simulink library "ROTH"  (R2016a)
settings: Solver=ode45  StartTime=0.0  StopTime=10.0  RelTol=1e-3
undefined symbols (not defined in the file): BUSY, CLEANED, EMPTY, FORWARD, GTSP, LEFT_BUSY_RIGHT_BUSY, LEFT_BUSY_RIGHT_CLEANED, LEFT_BUSY_RIGHT_EMPTY, LEFT_CLEANED_RIGHT_BUSY, LEFT_CLEANED_RIGHT_CLEANED, LEFT_CLEANED_RIGHT_EMPTY, LEFT_EMPTY_RIGHT_BUSY, LEFT_EMPTY_RIGHT_CLEANED, LEFT_EMPTY_RIGHT_EMPTY, MOVE_TURN_LEFT, MOVE_TURN_RIGHT, MOVE_U_TURN, MOVE_U_TURN_LEFT, MOVE_U_TURN_RIGHT, ROB_EAST, ROB_NORTH, ROB_SOUTH, ROB_WEST, STOP, UNCOVERED, ZIGZAG
settings Model: Creator=oelkawok  LastModifiedBy=oelkawok
settings DataIOCC: LimitDataPoints=on
settings DebuggingCC: AllowSymbolicDim=off

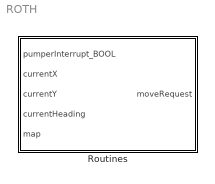
== system ROTH ==
  Routines : Subsystem

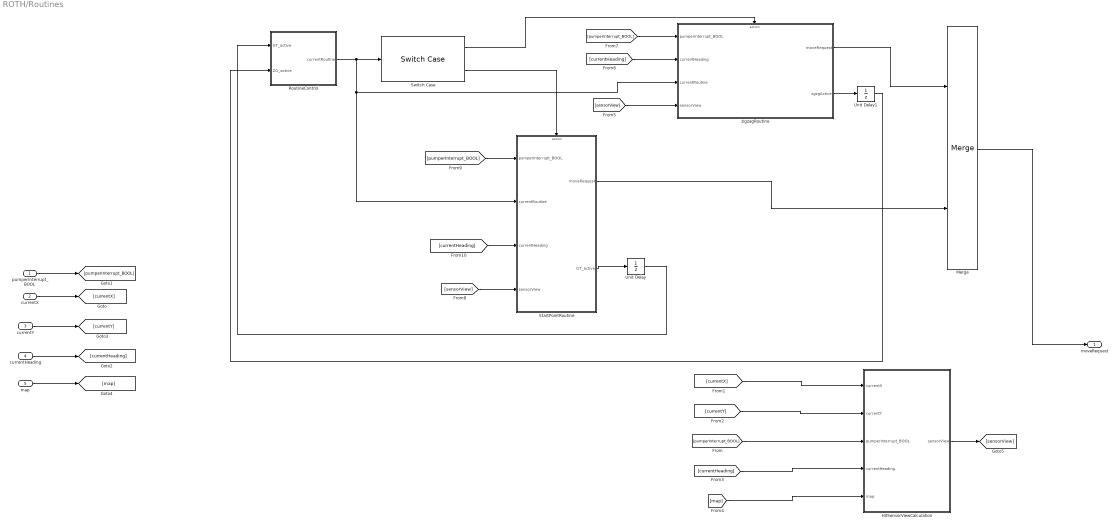
== system ROTH/Routines ==
  pumperInterrupt_BOOL : Inport
  currentX : Inport  Port=2
  currentY : Inport  Port=3
  currentHeading : Inport  Port=4
  map : Inport  Port=5
  HitSensorViewCalculation : Subsystem
  Merge : Merge
  RoutineControl : Subsystem
  StartPointRoutine : Subsystem
  Switch Case : SwitchCase  CaseConditions={ZIGZAG, GTSP}  ShowDefaultCase=off
      settings: AttributesFormatString=%<CaseConditions>
  Unit Delay : UnitDelay  InitialCondition=true  SampleTime=-1
  Unit Delay1 : UnitDelay  InitialCondition=false  SampleTime=-1
  zigzagRoutine : Subsystem
  moveRequest : Outport
  wires:
  [currentHeading] -> StartPointRoutine/3(currentHeading)
  [sensorView] -> StartPointRoutine/4(sensorView)
  [pumperInterrupt_BOOL] -> StartPointRoutine/1(pumperInterrupt_BOOL)
  Unit Delay1/1 -> RoutineControl/2(ZG_active)
  zigzagRoutine/2(zgzgActive) -> Unit Delay1/1
  zigzagRoutine/1(moveRequest) -> Merge/1
  StartPointRoutine/1(moveRequest) -> Merge/2
  [currentX] -> HitSensorViewCalculation/1(currentX)
  [currentY] -> HitSensorViewCalculation/2(currentY)
  [pumperInterrupt_BOOL] -> HitSensorViewCalculation/3(pumperInterrupt_BOOL)
  [currentHeading] -> HitSensorViewCalculation/4(currentHeading)
  [map] -> HitSensorViewCalculation/5(map)
  Switch Case/2 -> StartPointRoutine/Action
  Switch Case/1 -> zigzagRoutine/Action
  RoutineControl/1(currentRoutine) -> Switch Case/1, StartPointRoutine/2(currentRoutine), zigzagRoutine/3(currentRoutine)
  [currentHeading] -> zigzagRoutine/2(currentHeading)
  [pumperInterrupt_BOOL] -> zigzagRoutine/1(pumperInterrupt_BOOL)
  [sensorView] -> zigzagRoutine/4(sensorView)
  HitSensorViewCalculation/1(sensorView) -> [sensorView]
  Merge/1 -> moveRequest/1
  StartPointRoutine/2(GT_active) -> Unit Delay/1
  Unit Delay/1 -> RoutineControl/1(GT_active)
  pumperInterrupt_BOOL/1 -> [pumperInterrupt_BOOL]
  currentHeading/1 -> [currentHeading]
  currentY/1 -> [currentY]
  currentX/1 -> [currentX]
  map/1 -> [map]

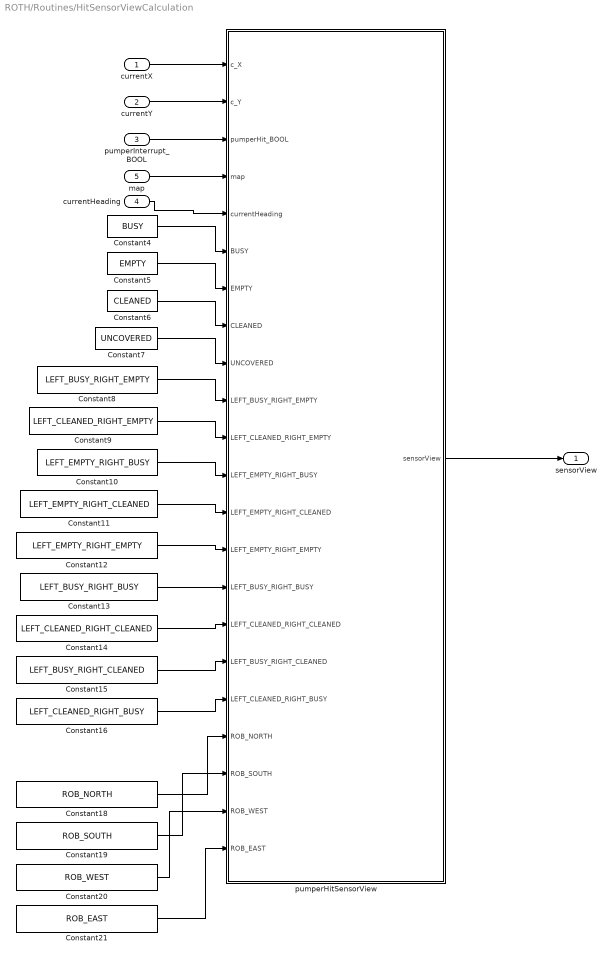
== system ROTH/Routines/HitSensorViewCalculation ==
  currentX : Inport
  currentY : Inport  Port=2
  pumperInterrupt_BOOL : Inport  Port=3
  currentHeading : Inport  Port=4
  map : Inport  Port=5
  Constant10 : Constant  Value=LEFT_EMPTY_RIGHT_BUSY
  Constant11 : Constant  Value=LEFT_EMPTY_RIGHT_CLEANED
  Constant12 : Constant  Value=LEFT_EMPTY_RIGHT_EMPTY
  Constant13 : Constant  Value=LEFT_BUSY_RIGHT_BUSY
  Constant14 : Constant  Value=LEFT_CLEANED_RIGHT_CLEANED
  Constant15 : Constant  Value=LEFT_BUSY_RIGHT_CLEANED
  Constant16 : Constant  Value=LEFT_CLEANED_RIGHT_BUSY
  Constant18 : Constant  Value=ROB_NORTH
  Constant19 : Constant  Value=ROB_SOUTH
  Constant20 : Constant  Value=ROB_WEST
  Constant21 : Constant  Value=ROB_EAST
  Constant4 : Constant  Value=BUSY
  Constant5 : Constant  Value=EMPTY
  Constant6 : Constant  Value=CLEANED
  Constant7 : Constant  Value=UNCOVERED
  Constant8 : Constant  Value=LEFT_BUSY_RIGHT_EMPTY
  Constant9 : Constant  Value=LEFT_CLEANED_RIGHT_EMPTY
  pumperHitSensorView : Stateflow chart  TreatAsAtomicUnit=on
  sensorView : Outport
  wires:
  Constant19/1 -> pumperHitSensorView/20(ROB_SOUTH)
  Constant21/1 -> pumperHitSensorView/22(ROB_EAST)
  Constant18/1 -> pumperHitSensorView/19(ROB_NORTH)
  Constant20/1 -> pumperHitSensorView/21(ROB_WEST)
  map/1 -> pumperHitSensorView/4(map)
  pumperInterrupt_BOOL/1 -> pumperHitSensorView/3(pumperHit_BOOL)
  currentX/1 -> pumperHitSensorView/1(c_X)
  currentY/1 -> pumperHitSensorView/2(c_Y)
  Constant8/1 -> pumperHitSensorView/10(LEFT_BUSY_RIGHT_EMPTY)
  Constant7/1 -> pumperHitSensorView/9(UNCOVERED)
  Constant5/1 -> pumperHitSensorView/7(EMPTY)
  Constant4/1 -> pumperHitSensorView/6(BUSY)
  Constant6/1 -> pumperHitSensorView/8(CLEANED)
  Constant10/1 -> pumperHitSensorView/12(LEFT_EMPTY_RIGHT_BUSY)
  Constant15/1 -> pumperHitSensorView/17(LEFT_BUSY_RIGHT_CLEANED)
  Constant12/1 -> pumperHitSensorView/14(LEFT_EMPTY_RIGHT_EMPTY)
  Constant13/1 -> pumperHitSensorView/15(LEFT_BUSY_RIGHT_BUSY)
  Constant9/1 -> pumperHitSensorView/11(LEFT_CLEANED_RIGHT_EMPTY)
  Constant11/1 -> pumperHitSensorView/13(LEFT_EMPTY_RIGHT_CLEANED)
  Constant14/1 -> pumperHitSensorView/16(LEFT_CLEANED_RIGHT_CLEANED)
  Constant16/1 -> pumperHitSensorView/18(LEFT_CLEANED_RIGHT_BUSY)
  pumperHitSensorView/1(sensorView) -> sensorView/1
  currentHeading/1 -> pumperHitSensorView/5(currentHeading)

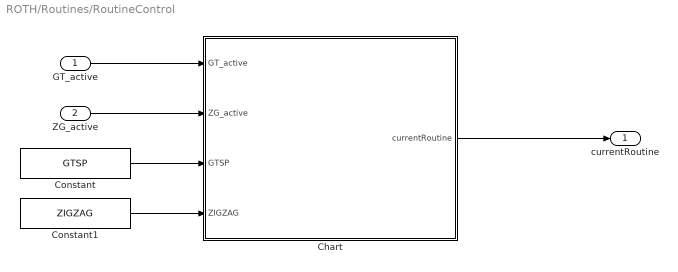
== system ROTH/Routines/RoutineControl ==
  GT_active : Inport
  ZG_active : Inport  Port=2
  Chart : Stateflow chart  TreatAsAtomicUnit=on
  Constant : Constant  Value=GTSP
  Constant1 : Constant  Value=ZIGZAG
  currentRoutine : Outport
  wires:
  ZG_active/1 -> Chart/2(ZG_active)
  GT_active/1 -> Chart/1(GT_active)
  Chart/1(currentRoutine) -> currentRoutine/1
  Constant/1 -> Chart/3(GTSP)
  Constant1/1 -> Chart/4(ZIGZAG)

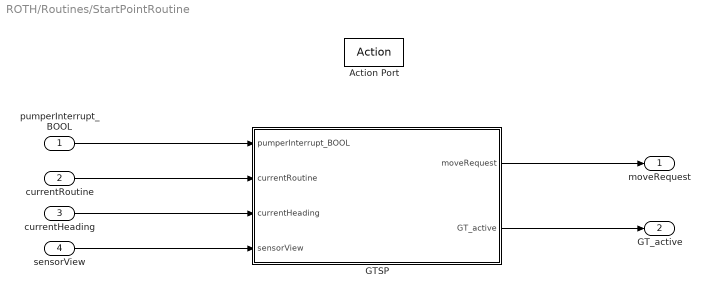
== system ROTH/Routines/StartPointRoutine ==
  pumperInterrupt_BOOL : Inport
  currentRoutine : Inport  Port=2
  currentHeading : Inport  Port=3
  sensorView : Inport  Port=4
  Action Port : ActionPort
  GTSP : Subsystem
  moveRequest : Outport
  GT_active : Outport  Port=2  InitialOutput=true
  wires:
  sensorView/1 -> GTSP/4(sensorView)
  pumperInterrupt_BOOL/1 -> GTSP/1(pumperInterrupt_BOOL)
  currentRoutine/1 -> GTSP/2(currentRoutine)
  currentHeading/1 -> GTSP/3(currentHeading)
  GTSP/1(moveRequest) -> moveRequest/1
  GTSP/2(GT_active) -> GT_active/1

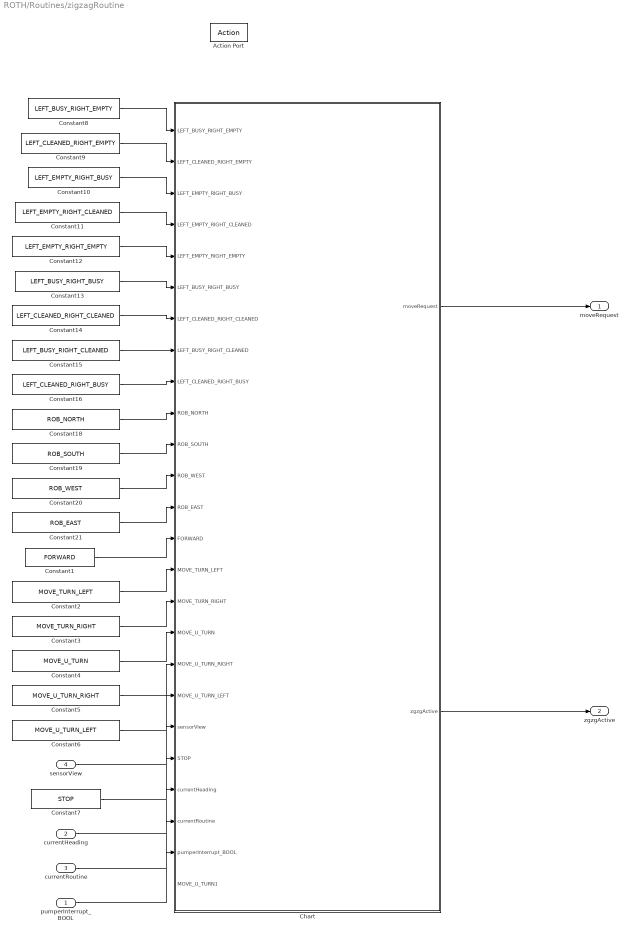
== system ROTH/Routines/zigzagRoutine ==
  pumperInterrupt_BOOL : Inport
  currentHeading : Inport  Port=2
  currentRoutine : Inport  Port=3
  sensorView : Inport  Port=4
  Action Port : ActionPort
  Chart : Stateflow chart  TreatAsAtomicUnit=on
  Constant1 : Constant  Value=FORWARD
  Constant10 : Constant  Value=LEFT_EMPTY_RIGHT_BUSY
  Constant11 : Constant  Value=LEFT_EMPTY_RIGHT_CLEANED
  Constant12 : Constant  Value=LEFT_EMPTY_RIGHT_EMPTY
  Constant13 : Constant  Value=LEFT_BUSY_RIGHT_BUSY
  Constant14 : Constant  Value=LEFT_CLEANED_RIGHT_CLEANED
  Constant15 : Constant  Value=LEFT_BUSY_RIGHT_CLEANED
  Constant16 : Constant  Value=LEFT_CLEANED_RIGHT_BUSY
  Constant18 : Constant  Value=ROB_NORTH
  Constant19 : Constant  Value=ROB_SOUTH
  Constant2 : Constant  Value=MOVE_TURN_LEFT
  Constant20 : Constant  Value=ROB_WEST
  Constant21 : Constant  Value=ROB_EAST
  Constant3 : Constant  Value=MOVE_TURN_RIGHT
  Constant4 : Constant  Value=MOVE_U_TURN
  Constant5 : Constant  Value=MOVE_U_TURN_RIGHT
  Constant6 : Constant  Value=MOVE_U_TURN_LEFT
  Constant7 : Constant  Value=STOP
  Constant8 : Constant  Value=LEFT_BUSY_RIGHT_EMPTY
  Constant9 : Constant  Value=LEFT_CLEANED_RIGHT_EMPTY
  moveRequest : Outport
  zgzgActive : Outport  Port=2
  wires:
  Chart/2(zgzgActive) -> zgzgActive/1
  Chart/1(moveRequest) -> moveRequest/1
  Constant7/1 -> Chart/21(STOP)
  currentHeading/1 -> Chart/22(currentHeading)
  currentRoutine/1 -> Chart/23(currentRoutine)
  sensorView/1 -> Chart/20(sensorView)
  pumperInterrupt_BOOL/1 -> Chart/24(pumperInterrupt_BOOL)
  Constant5/1 -> Chart/18(MOVE_U_TURN_RIGHT)
  Constant6/1 -> Chart/19(MOVE_U_TURN_LEFT)
  Constant2/1 -> Chart/15(MOVE_TURN_LEFT)
  Constant3/1 -> Chart/16(MOVE_TURN_RIGHT)
  Constant4/1 -> Chart/17(MOVE_U_TURN)
  Constant1/1 -> Chart/14(FORWARD)
  Constant16/1 -> Chart/9(LEFT_CLEANED_RIGHT_BUSY)
  Constant10/1 -> Chart/3(LEFT_EMPTY_RIGHT_BUSY)
  Constant12/1 -> Chart/5(LEFT_EMPTY_RIGHT_EMPTY)
  Constant11/1 -> Chart/4(LEFT_EMPTY_RIGHT_CLEANED)
  Constant14/1 -> Chart/7(LEFT_CLEANED_RIGHT_CLEANED)
  Constant19/1 -> Chart/11(ROB_SOUTH)
  Constant18/1 -> Chart/10(ROB_NORTH)
  Constant15/1 -> Chart/8(LEFT_BUSY_RIGHT_CLEANED)
  Constant13/1 -> Chart/6(LEFT_BUSY_RIGHT_BUSY)
  Constant20/1 -> Chart/12(ROB_WEST)
  Constant9/1 -> Chart/2(LEFT_CLEANED_RIGHT_EMPTY)
  Constant8/1 -> Chart/1(LEFT_BUSY_RIGHT_EMPTY)
  Constant21/1 -> Chart/13(ROB_EAST)

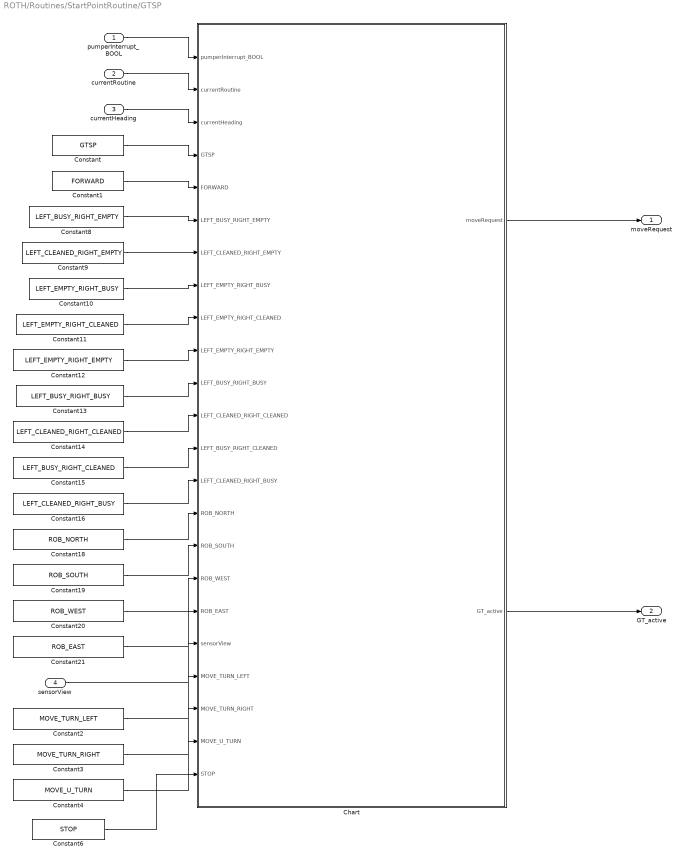
== system ROTH/Routines/StartPointRoutine/GTSP ==
  pumperInterrupt_BOOL : Inport
  currentRoutine : Inport  Port=2
  currentHeading : Inport  Port=3
  sensorView : Inport  Port=4
  Chart : Stateflow chart  TreatAsAtomicUnit=on
  Constant : Constant  Value=GTSP
  Constant1 : Constant  Value=FORWARD
  Constant10 : Constant  Value=LEFT_EMPTY_RIGHT_BUSY
  Constant11 : Constant  Value=LEFT_EMPTY_RIGHT_CLEANED
  Constant12 : Constant  Value=LEFT_EMPTY_RIGHT_EMPTY
  Constant13 : Constant  Value=LEFT_BUSY_RIGHT_BUSY
  Constant14 : Constant  Value=LEFT_CLEANED_RIGHT_CLEANED
  Constant15 : Constant  Value=LEFT_BUSY_RIGHT_CLEANED
  Constant16 : Constant  Value=LEFT_CLEANED_RIGHT_BUSY
  Constant18 : Constant  Value=ROB_NORTH
  Constant19 : Constant  Value=ROB_SOUTH
  Constant2 : Constant  Value=MOVE_TURN_LEFT
  Constant20 : Constant  Value=ROB_WEST
  Constant21 : Constant  Value=ROB_EAST
  Constant3 : Constant  Value=MOVE_TURN_RIGHT
  Constant4 : Constant  Value=MOVE_U_TURN
  Constant6 : Constant  Value=STOP
  Constant8 : Constant  Value=LEFT_BUSY_RIGHT_EMPTY
  Constant9 : Constant  Value=LEFT_CLEANED_RIGHT_EMPTY
  moveRequest : Outport
  GT_active : Outport  Port=2
  wires:
  currentHeading/1 -> Chart/3(currentHeading)
  pumperInterrupt_BOOL/1 -> Chart/1(pumperInterrupt_BOOL)
  currentRoutine/1 -> Chart/2(currentRoutine)
  Constant/1 -> Chart/4(GTSP)
  Constant1/1 -> Chart/5(FORWARD)
  Constant8/1 -> Chart/6(LEFT_BUSY_RIGHT_EMPTY)
  Constant9/1 -> Chart/7(LEFT_CLEANED_RIGHT_EMPTY)
  Constant10/1 -> Chart/8(LEFT_EMPTY_RIGHT_BUSY)
  Constant11/1 -> Chart/9(LEFT_EMPTY_RIGHT_CLEANED)
  Constant12/1 -> Chart/10(LEFT_EMPTY_RIGHT_EMPTY)
  Constant13/1 -> Chart/11(LEFT_BUSY_RIGHT_BUSY)
  Constant14/1 -> Chart/12(LEFT_CLEANED_RIGHT_CLEANED)
  Constant15/1 -> Chart/13(LEFT_BUSY_RIGHT_CLEANED)
  Constant16/1 -> Chart/14(LEFT_CLEANED_RIGHT_BUSY)
  Constant21/1 -> Chart/18(ROB_EAST)
  Constant20/1 -> Chart/17(ROB_WEST)
  Constant19/1 -> Chart/16(ROB_SOUTH)
  Constant18/1 -> Chart/15(ROB_NORTH)
  sensorView/1 -> Chart/19(sensorView)
  Constant4/1 -> Chart/22(MOVE_U_TURN)
  Constant3/1 -> Chart/21(MOVE_TURN_RIGHT)
  Constant2/1 -> Chart/20(MOVE_TURN_LEFT)
  Chart/1(moveRequest) -> moveRequest/1
  Chart/2(GT_active) -> GT_active/1
  Constant6/1 -> Chart/23(STOP)

== stateflow chart ROTH/Routines/HitSensorViewCalculation/pumperHitSensorView ==
  state SensorViewState
  state Init
    entry:
    sensorView = 0;
  state NoHit
    entry:
    currentY = c_Y - 1;
    currentX = c_X - 1;
  (junction 10) -> SensorViewState [order 1] : [(map[currentY][currentX - 1] == BUSY) ...
      | && ( (map[currentY][currentX + 1] == EMPTY)...
      |  || (map[currentY][currentX+1] == UNCOVERED) )]...
      | /sensorView = LEFT_BUSY_RIGHT_EMPTY;
  (junction 10) -> SensorViewState [order 2] : [(map[currentY][currentX - 1] == CLEANED) ...
      | && ((map[currentY][currentX + 1] == EMPTY)...
      | || (map[currentY][currentX+1] == UNCOVERED))]
      | /{sensorView =  LEFT_CLEANED_RIGHT_EMPTY;}
  (junction 10) -> SensorViewState [order 3] : [((map[currentY][currentX - 1] == EMPTY) ...
      | || (map[currentY][currentX - 1] == UNCOVERED))...
      | && (map[currentY][currentX + 1] == BUSY)]
      | /{sensorView = LEFT_EMPTY_RIGHT_BUSY;}
  (junction 10) -> SensorViewState [order 4] : [(map[currentY][currentX + 1] == CLEANED) ...
      | && ((map[currentY][currentX - 1] == EMPTY)...
      | || (map[currentY][currentX - 1] == UNCOVERED))]
      | /{sensorView =  LEFT_EMPTY_RIGHT_CLEANED;}
  (junction 10) -> SensorViewState [order 5] : [((map[currentY][currentX + 1] == EMPTY) ...
      | || (map[currentY][currentX + 1] == UNCOVERED))...
      | && ((map[currentY][currentX - 1] == EMPTY)...
      | || (map[currentY][currentX - 1] == UNCOVERED))]
      | /{sensorView = LEFT_EMPTY_RIGHT_EMPTY;}
  (junction 10) -> SensorViewState [order 6] : [(map[currentY][currentX - 1] == BUSY) ...
      | && (map[currentY][currentX + 1] == BUSY)]
      | /{sensorView = LEFT_BUSY_RIGHT_BUSY;}
  (junction 10) -> SensorViewState [order 7] : [(map[currentY][currentX - 1] == CLEANED) ...
      | && (map[currentY][currentX + 1] == CLEANED)]
      | /{sensorView = LEFT_CLEANED_RIGHT_CLEANED;}
  (junction 10) -> SensorViewState [order 8] : [(map[currentY][currentX - 1] == BUSY) ...
      | && (map[currentY][currentX + 1] == CLEANED)]
      | /{sensorView = LEFT_BUSY_RIGHT_CLEANED;}
  (junction 10) -> SensorViewState [order 9] : [(map[currentY][currentX - 1] == CLEANED) ...
      | && (map[currentY][currentX + 1] == BUSY)]
      | /{sensorView = LEFT_CLEANED_RIGHT_BUSY;}
  (junction 8) -> (junction 10) [order 1] : [currentHeading == ROB_NORTH]
  (default) -> Init
  (junction 11) -> SensorViewState [order 2] : [(map[currentY][currentX - 1] == BUSY) ...
      | && ( (map[currentY][currentX + 1] == EMPTY)...
      |  || (map[currentY][currentX+1] == UNCOVERED) )]...
      | /sensorView = LEFT_EMPTY_RIGHT_BUSY;
  Init -> NoHit
  NoHit -> (junction 8) : [pumperHit_BOOL]
  (junction 8) -> (junction 15) [order 4] : [currentHeading == ROB_EAST]
  (junction 8) -> (junction 13) [order 3] : [currentHeading == ROB_WEST]
  (junction 8) -> (junction 11) [order 2] : [currentHeading == ROB_SOUTH]
  SensorViewState -> NoHit
  (junction 11) -> SensorViewState [order 1] : [(map[currentY][currentX - 1] == CLEANED) ...
      | && ((map[currentY][currentX + 1] == EMPTY)...
      | || (map[currentY][currentX+1] == UNCOVERED))]
      | /{sensorView =  LEFT_EMPTY_RIGHT_CLEANED;}
  (junction 11) -> SensorViewState [order 5] : [((map[currentY][currentX - 1] == EMPTY) ...
      | || (map[currentY][currentX - 1] == UNCOVERED))...
      | && (map[currentY][currentX + 1] == BUSY)]
      | /{sensorView = LEFT_BUSY_RIGHT_EMPTY;}
  (junction 11) -> SensorViewState [order 6] : [(map[currentY][currentX + 1] == CLEANED) ...
      | && ((map[currentY][currentX - 1] == EMPTY)...
      | || (map[currentY][currentX - 1] == UNCOVERED))]
      | /{sensorView =  LEFT_CLEANED_RIGHT_EMPTY;}
  (junction 11) -> SensorViewState [order 4] : [((map[currentY][currentX + 1] == EMPTY) ...
      | || (map[currentY][currentX + 1] == UNCOVERED))...
      | && ((map[currentY][currentX - 1] == EMPTY)...
      | || (map[currentY][currentX - 1] == UNCOVERED))]
      | /{sensorView = LEFT_EMPTY_RIGHT_EMPTY;}
  (junction 11) -> SensorViewState [order 8] : [(map[currentY][currentX - 1] == BUSY) ...
      | && (map[currentY][currentX + 1] == CLEANED)]
      | /{sensorView = LEFT_CLEANED_RIGHT_BUSY;}
  (junction 11) -> SensorViewState [order 3] : [(map[currentY][currentX - 1] == BUSY) ...
      | && (map[currentY][currentX + 1] == BUSY)]
      | /{sensorView = LEFT_BUSY_RIGHT_BUSY;}
  (junction 11) -> SensorViewState [order 7] : [(map[currentY][currentX - 1] == CLEANED) ...
      | && (map[currentY][currentX + 1] == CLEANED)]
      | /{sensorView = LEFT_CLEANED_RIGHT_CLEANED;}
  (junction 11) -> SensorViewState [order 9] : [(map[currentY][currentX - 1] == CLEANED) ...
      | && (map[currentY][currentX + 1] == BUSY)]
      | /{sensorView = LEFT_BUSY_RIGHT_CLEANED;}
  data: c_X input; c_Y input; pumperHit_BOOL input; sensorView output uint8; map input size=[ROOM_SIDE_SIZE ROOM_SIDE_SIZE]; currentHeading input; BUSY input; EMPTY input; CLEANED input; UNCOVERED input; LEFT_BUSY_RIGHT_EMPTY input; LEFT_CLEANED_RIGHT_EMPTY input; LEFT_EMPTY_RIGHT_BUSY input; LEFT_EMPTY_RIGHT_CLEANED input; LEFT_EMPTY_RIGHT_EMPTY input; LEFT_BUSY_RIGHT_BUSY input; LEFT_CLEANED_RIGHT_CLEANED input; LEFT_BUSY_RIGHT_CLEANED input; LEFT_CLEANED_RIGHT_BUSY input; ROB_NORTH input; ROB_SOUTH input; ROB_WEST input; ROB_EAST input; currentX local uint8; currentY local uint8

== stateflow chart ROTH/Routines/zigzagRoutine/Chart ==
  state SwitchLane
  state finishZigZag
    en:
    zgzgActive = false;
  state Idle
  state MovingForward
    en:
    moveRequest = FORWARD;
  (junction 34) -> SwitchLane [order 1] : [currentHeading == ROB_NORTH]
      | /moveRequest = MOVE_U_TURN_RIGHT;
      | headingRequest = ROB_SOUTH;
  (junction 34) -> SwitchLane [order 2] : [currentHeading == ROB_SOUTH]
      | /moveRequest = MOVE_U_TURN_LEFT;
      | headingRequest = ROB_NORTH;
  (junction 35) -> SwitchLane [order 1] : [currentHeading == ROB_NORTH]
      | /moveRequest = MOVE_U_TURN_RIGHT;
      | headingRequest = ROB_SOUTH;
  (junction 33) -> (junction 34) [order 1] : [sensorView == LEFT_EMPTY_RIGHT_EMPTY]
  SwitchLane -> finishZigZag [order 1] : [finishCounter > 2]
  (junction 35) -> SwitchLane [order 2] : [currentHeading == ROB_SOUTH]
      | /moveRequest = MOVE_U_TURN;
      | headingRequest = ROB_NORTH;
  (junction 33) -> (junction 35) [order 2] : [(sensorView == LEFT_CLEANED_RIGHT_EMPTY)...
      | || (sensorView == LEFT_BUSY_RIGHT_EMPTY)]
  (junction 36) -> SwitchLane [order 2] : [currentHeading == ROB_SOUTH]
      | /moveRequest = MOVE_U_TURN_LEFT;
      | headingRequest = ROB_NORTH;
  (default) -> Idle
  Idle -> MovingForward : [currentRoutine == ZIGZAG]
      | /zgzgActive = true;
  MovingForward -> (junction 33) : [pumperInterrupt_BOOL]
      | /moveRequest = STOP;
  (junction 36) -> SwitchLane [order 1] : [currentHeading == ROB_NORTH]
      | /moveRequest = MOVE_U_TURN;
      | headingRequest = ROB_SOUTH;
  (junction 33) -> (junction 36) [order 3] : [(sensorView == LEFT_EMPTY_RIGHT_CLEANED)...
      | || (sensorView == LEFT_EMPTY_RIGHT_BUSY)]
  (junction 33) -> (junction 37) [order 4] : [(sensorView == LEFT_BUSY_RIGHT_BUSY)...
      | || (sensorView == LEFT_BUSY_RIGHT_CLEANED)...
      | || (sensorView == LEFT_CLEANED_RIGHT_BUSY)...
      | || (sensorView == LEFT_CLEANED_RIGHT_CLEANED)]
  SwitchLane -> MovingForward [order 2] : [headingRequest == currentHeading]
  (junction 37) -> SwitchLane [order 1] : [currentHeading == ROB_NORTH]
      | /moveRequest = MOVE_U_TURN;
      | headingRequest = ROB_SOUTH;
      | finishCounter++;
  (junction 37) -> SwitchLane [order 2] : [currentHeading == ROB_SOUTH]
      | /moveRequest = MOVE_U_TURN;
      | headingRequest = ROB_NORTH;
      | finishCounter++;
  data: LEFT_BUSY_RIGHT_EMPTY input; LEFT_CLEANED_RIGHT_EMPTY input; LEFT_EMPTY_RIGHT_BUSY input; LEFT_EMPTY_RIGHT_CLEANED input; LEFT_EMPTY_RIGHT_EMPTY input; LEFT_BUSY_RIGHT_BUSY input; LEFT_CLEANED_RIGHT_CLEANED input; LEFT_BUSY_RIGHT_CLEANED input; LEFT_CLEANED_RIGHT_BUSY input; ROB_NORTH input; ROB_SOUTH input; ROB_WEST input; ROB_EAST input; FORWARD input; MOVE_TURN_LEFT input; MOVE_TURN_RIGHT input; MOVE_U_TURN input; MOVE_U_TURN_RIGHT input; MOVE_U_TURN_LEFT input; sensorView input; STOP input; moveRequest output uint8; currentHeading input; currentRoutine input; pumperInterrupt_BOOL input; MOVE_U_TURN1 input; headingRequest local double; ZIGZAG parameter; zgzgActive output boolean; finishCounter local uint8

== stateflow chart ROTH/Routines/StartPointRoutine/GTSP/Chart ==
  state GTSP_Active
    state Forward
      entry:
      moveRequest = FORWARD;
    state TurnLeft
      entry:
      moveRequest = MOVE_TURN_LEFT;
    state preFinishLeftBlockedN
      entry:
      moveRequest = MOVE_U_TURN;
    state preFinishLeftBlockedW
      entry:
      moveRequest = MOVE_TURN_RIGHT;
    state preFinishNormal
      entry:
      moveRequest = MOVE_TURN_LEFT;
    state preFinishBlockedW
    state preFinishBlockedN
      entry:
      moveRequest = MOVE_U_TURN;
    state finishedGTSP
      entry:
      moveRequest = STOP;
      GT_active = false;
    TurnLeft -> Forward : [currentHeading == ROB_WEST]
    (default) -> Forward
    Forward -> (junction 14) : [pumperInterrupt_BOOL]
        | /moveRequest = STOP;
    (junction 14) -> (junction 17) [order 1] : [(sensorView == LEFT_EMPTY_RIGHT_EMPTY)...
        | || (sensorView == LEFT_EMPTY_RIGHT_CLEANED)...
        | || (sensorView == LEFT_EMPTY_RIGHT_BUSY)]
    (junction 14) -> (junction 22) [order 2] : [(sensorView == LEFT_CLEANED_RIGHT_EMPTY)...
        | || (sensorView == LEFT_BUSY_RIGHT_EMPTY)]
    (junction 14) -> (junction 29) [order 3] : [(sensorView == LEFT_BUSY_RIGHT_BUSY)...
        | || (sensorView == LEFT_BUSY_RIGHT_CLEANED)...
        | || (sensorView == LEFT_CLEANED_RIGHT_BUSY)...
        | || (sensorView == LEFT_CLEANED_RIGHT_CLEANED)]
    (junction 17) -> TurnLeft [order 1] : [currentHeading == ROB_NORTH]
    (junction 17) -> preFinishNormal [order 2] : [currentHeading == ROB_WEST]
    (junction 22) -> preFinishLeftBlockedW [order 2] : [currentHeading == ROB_WEST]
    (junction 22) -> preFinishLeftBlockedN [order 1] : [currentHeading == ROB_NORTH]
    (junction 29) -> preFinishBlockedW [order 1] : [currentHeading == ROB_WEST]
    (junction 29) -> preFinishBlockedN [order 2] : [currentHeading == ROB_NORTH]
    preFinishLeftBlockedN -> finishedGTSP : [currentHeading == ROB_SOUTH]
    preFinishLeftBlockedW -> finishedGTSP : [currentHeading == ROB_NORTH]
    preFinishNormal -> finishedGTSP : [currentHeading == ROB_SOUTH]
    preFinishBlockedN -> finishedGTSP : [currentHeading == ROB_NORTH]
    preFinishBlockedW -> finishedGTSP
  state Idle
  (default) -> Idle
  Idle -> GTSP_Active : [currentRoutine == GTSP]
      | /GT_active = true;
  GTSP_Active -> Idle : [currentRoutine != GTSP]
  data: pumperInterrupt_BOOL input; currentRoutine input; currentHeading input; GTSP input; FORWARD input; LEFT_BUSY_RIGHT_EMPTY input; LEFT_CLEANED_RIGHT_EMPTY input; LEFT_EMPTY_RIGHT_BUSY input; LEFT_EMPTY_RIGHT_CLEANED input; LEFT_EMPTY_RIGHT_EMPTY input; LEFT_BUSY_RIGHT_BUSY input; LEFT_CLEANED_RIGHT_CLEANED input; LEFT_BUSY_RIGHT_CLEANED input; LEFT_CLEANED_RIGHT_BUSY input; ROB_NORTH input; ROB_SOUTH input; ROB_WEST input; ROB_EAST input; sensorView input; moveRequest output uint8; MOVE_TURN_LEFT input; MOVE_TURN_RIGHT input; MOVE_U_TURN input; GT_active output boolean =true; STOP input

== stateflow chart ROTH/Routines/RoutineControl/Chart ==
  state GTSP
    entry:
    currentRoutine = GTSP;
  state init
  state ZIGZAG
    entry:
    currentRoutine = ZIGZAG;
  state End
  (default) -> init
  GTSP -> ZIGZAG : [GT_active == false]
  init -> GTSP
  ZIGZAG -> End : [ZG_active == false]
  data: currentRoutine output uint8; GT_active input; ZG_active input; GTSP input; ZIGZAG input
